simulink model "predatorprey"  (R2017a)
settings: Solver=FixedStepAuto  StartTime=1  StopTime=40  FixedStep=0.1  RelTol=1e-3
model workspace (MAT data in the model file):
  D0 = 1
  P0 = 2.95
  beta = 0.5
  delta = 0.5
  ro = 2.5
settings Model: Creator=Usuario  LastModifiedBy=drojasd
settings DataIOCC: SaveFormat=Array  ReturnWorkspaceOutputs=on  OutputTimes=tout

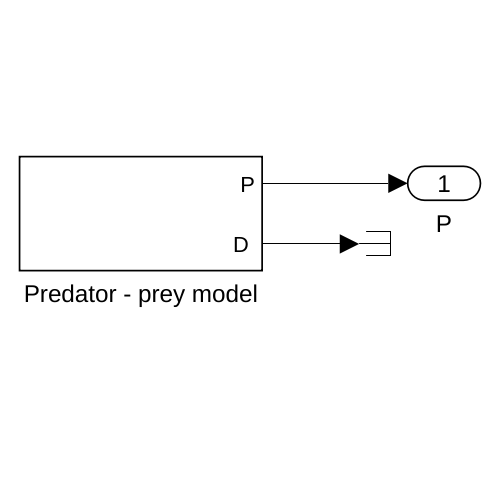
[thumbnail: Simulink's stored preview of the top-level diagram]
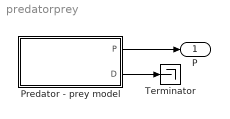
== system predatorprey ==
  "Predator - prey model " : Subsystem  mask{delta=delta, beta=beta, ro=ro, P0=P0, D0=D0}
  Terminator : Terminator
  P : Outport
  wires:
  "Predator - prey model "/1(P) -> P/1
  "Predator - prey model "/2("D ") -> Terminator/1

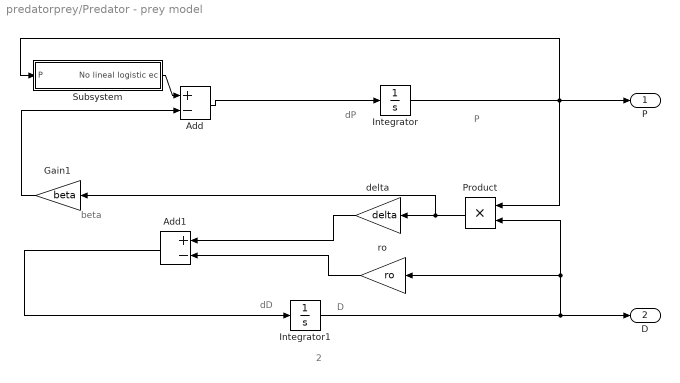
== system predatorprey/Predator - prey model  ==
  note: 2
  note: beta
  note: D
  note: dD
  note: dP
  note: P
  Add : Sum  Inputs=+-
  Add1 : Sum  Inputs=+-
  Gain1 : Gain  Gain=beta
  Integrator : Integrator  InitialCondition=P0
  Integrator1 : Integrator  InitialCondition=D0
  Product : Product
  Subsystem : Subsystem
  delta : Gain  Gain=delta
  ro : Gain  Gain=ro
  P : Outport
  "D " : Outport  Port=2
  wires:
  Add/1 -> Integrator/1
  delta/1 -> Add1/1
  Integrator/1 -> Product/1, P/1, Subsystem/1(P)
  Add1/1 -> Integrator1/1
  Gain1/1 -> Add/2
  Integrator1/1 -> Product/2, ro/1, "D "/1
  ro/1 -> Add1/2
  Product/1 -> Gain1/1, delta/1
  Subsystem/1("No lineal logistic ec ") -> Add/1

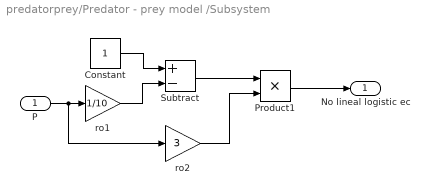
== system predatorprey/Predator - prey model /Subsystem ==
  P : Inport
  Constant : Constant
  Product1 : Product
  Subtract : Sum  Inputs=+-
  ro1 : Gain  Gain=1/10
  ro2 : Gain  Gain=3
  "No lineal logistic ec " : Outport
  wires:
  Subtract/1 -> Product1/1
  ro2/1 -> Product1/2
  Product1/1 -> "No lineal logistic ec "/1
  Constant/1 -> Subtract/1
  P/1 -> ro2/1, ro1/1
  ro1/1 -> Subtract/2
